simulink model "Parkhaus_inherited"  (Simulink 4.00)
settings: Solver=FixedStepDiscrete  StartTime=0.0  StopTime=1000000000  FixedStep=0.001  RelTol=1e-3
libraries: simulink3 x2
settings Model: LastModifiedBy=Administrator  BlockReductionOpt=off

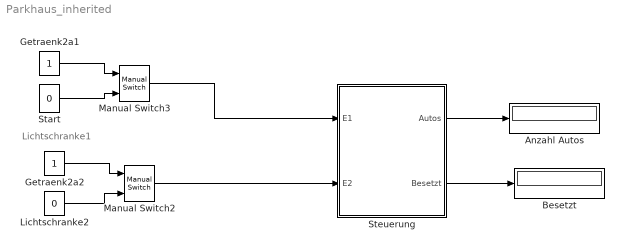
== system Parkhaus_inherited ==
  note: Lichtschranke1
  Anzahl Autos : Display
      settings: Format=short
  Besetzt : Display
      settings: Format=short
  Getraenk2a1 : Constant  Value=1
  Getraenk2a2 : Constant  Value=1
  Lichtschranke2 : Constant  Value=0
  Manual Switch2 : simulink3/Nonlinear/Manual Switch  sw=0  action=0
  Manual Switch3 : simulink3/Nonlinear/Manual Switch  sw=0  action=0
  Start : Constant  Value=0
  Steuerung : Stateflow chart  TreatAsAtomicUnit=on
      settings: RTWFcnNameOpts=Auto  RTWFileNameOpts=Auto
  wires:
  Start/1 -> Manual Switch3/2
  Manual Switch3/1 -> Steuerung/1(E1)
  Steuerung/1(Autos) -> Anzahl Autos/1
  Getraenk2a1/1 -> Manual Switch3/1
  Steuerung/2(Besetzt) -> Besetzt/1
  Lichtschranke2/1 -> Manual Switch2/2
  Getraenk2a2/1 -> Manual Switch2/1
  Manual Switch2/1 -> Steuerung/2(E2)

== stateflow chart Steuerung ==
  state Idle
    entry:
    Besetzt=ml('parkhaus(%d,%d)',Autos,Plaetze)
  state ZE1
  state ZA3
  state ZE2
  state ZE3
  state ZA1
  state ZA2
  (default) -> Idle
  Idle -> ZE1 : [E1==1 & E2==0]
  Idle -> ZA1 : [E1==0 & E2==1]
  ZE1 -> ZE2 : [E1==1 & E2==1]
  ZE1 -> Idle : [E1==0 & E2==0]
  ZA1 -> Idle : [E1==0 & E2==0]
  ZA1 -> ZA2 : [E1==1 & E2==1]
  ZA2 -> ZA3 : [E1==1 & E2==0]
  ZE3 -> Idle : [E1==0 & E2==0]/Autos++;
  ZE2 -> ZE1 : [E1==1 & E2==0]
  ZA2 -> ZA1 : [E1==0 & E2==1]
  ZA3 -> ZA2 : [E1==1 & E2==1]
  ZE2 -> ZE3 : [E1==0 & E2==1]
  ZE3 -> ZE2 : [E1==1 & E2==0]
  ZA3 -> Idle : [E1==0 & E2==0]/Autos--
  data: E1 input boolean; E2 input boolean; Autos output int16; Besetzt output int16; Plaetze constant int16 =5
